simulink model "BD_INTERACTIVE_REPLAY"  (Simulink 4.00)
settings: Solver=FixedStepDiscrete  StartTime=0.0  StopTime=inf  FixedStep=1  RelTol=1e-3
undefined symbols (not defined in the file): fc_plot_axis, mc_plot_axis
libraries: lib_interactive x1
settings Model: LastModifiedBy=mokeefe  LimitDataPoints=off  ExtModeTrigMode=oneshot  ExtModeArmWhenConnect=off
settings Model: ModifiedComment=|
  | mokeefe -- Thu Apr 18 07:59:04 2002 -- Version 1.86
  | saving the model:
  | o "without the model browser open"
  | o with only top-level screen visible
  | o and with "fit to view" enabled
settings Model: ModifiedHistory=|
  | mokeefe -- Thu Apr 18 07:59:04 2002 -- Version 1.86
  | saving the model:
  | o "without the model browser open"
  | o with only top-level screen visible
  | o and with "fit to view" enabled

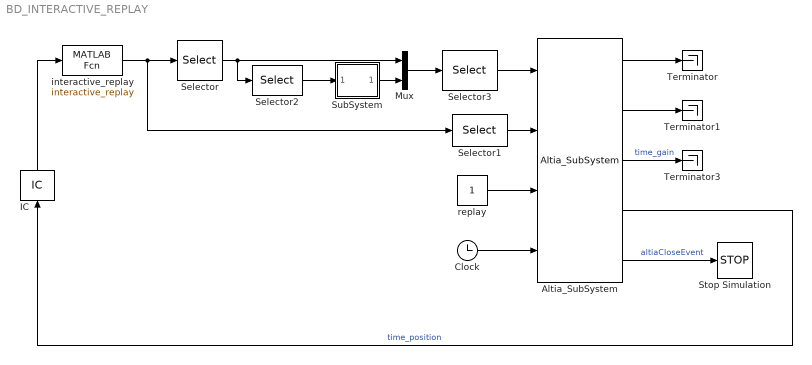
== system BD_INTERACTIVE_REPLAY ==
  Altia_SubSystem : lib_interactive/Altia_SubSystem
      settings: RTWFcnNameOpts=Auto  RTWFileNameOpts=Auto
  Clock : Clock
      settings: DisplayTime=off  Decimation=10
  IC : InitialCondition  Orientation=up  Value=1
  Mux : Mux  Inputs=2
  Selector : Selector  InputType=Vector  ElementSrc=Internal  Elements=[2:47 60 49:59]  RowSrc=Internal  Rows=1  ColumnSrc=Internal  Columns=1  InputPortWidth=60
  Selector1 : Selector  InputType=Vector  ElementSrc=Internal  Elements=[1]  RowSrc=Internal  Rows=1  ColumnSrc=Internal  Columns=1  InputPortWidth=60
  Selector2 : Selector  InputType=Vector  ElementSrc=Internal  Elements=[22 23 56 57 58]  RowSrc=Internal  Rows=1  ColumnSrc=Internal  Columns=1  InputPortWidth=58
  Selector3 : Selector  InputType=Vector  ElementSrc=Internal  Elements=[1:28 59 60 31:52 61 62 63 56:58]  RowSrc=Internal  Rows=1  ColumnSrc=Internal  Columns=1  InputPortWidth=63
  Stop Simulation : Stop
  SubSystem : Subsystem
      settings: RTWFcnNameOpts=Auto  RTWFileNameOpts=Auto
  Terminator : Terminator
  Terminator1 : Terminator
  Terminator3 : Terminator
  interactive_replay : MATLABFcn  MATLABFcn=interactive_replay  OutputDimensions=60  OutputSignalType=auto  Output1D=on
  replay : Constant  Value=1
  wires:
  interactive_replay/1 -> Selector/1, Selector1/1
  Altia_SubSystem/1 -> Terminator/1
  Altia_SubSystem/2 -> Terminator1/1
  replay/1 -> Altia_SubSystem/3
  Altia_SubSystem/3 -> Terminator3/1  "time_gain"
  Clock/1 -> Altia_SubSystem/4
  Altia_SubSystem/5 -> Stop Simulation/1  "altiaCloseEvent"
  Selector1/1 -> Altia_SubSystem/2
  Selector3/1 -> Altia_SubSystem/1
  Selector/1 -> Selector2/1, Mux/1
  Mux/1 -> Selector3/1
  Selector2/1 -> SubSystem/1(In1)
  SubSystem/1(Out1) -> Mux/2
  IC/1 -> interactive_replay/1
  Altia_SubSystem/4 -> IC/1  "time_position"

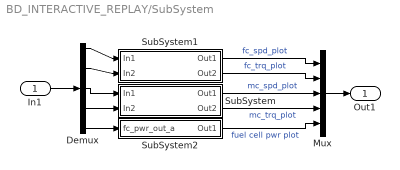
== system BD_INTERACTIVE_REPLAY/SubSystem ==
  In1 : Inport  Port=1  LatchInput=off
  Demux : Demux  Outputs=5  BusSelectionMode=off
  Mux : Mux  Inputs=5
  SubSystem : Subsystem
      settings: RTWFcnNameOpts=Auto  RTWFileNameOpts=Auto
  SubSystem1 : Subsystem
      settings: RTWFcnNameOpts=Auto  RTWFileNameOpts=Auto
  SubSystem2 : Subsystem
      settings: RTWFcnNameOpts=Auto  RTWFileNameOpts=Auto
  Out1 : Outport  Port=1
  wires:
  In1/1 -> Demux/1
  Demux/1 -> SubSystem1/1(In1)
  Demux/2 -> SubSystem1/2(In2)
  Demux/3 -> SubSystem/1(In1)
  Demux/4 -> SubSystem/2(In2)
  SubSystem/1(Out1) -> Mux/3  "mc_spd_plot"
  SubSystem/2(Out2) -> Mux/4  "mc_trq_plot"
  SubSystem1/1(Out1) -> Mux/1  "fc_spd_plot"
  SubSystem1/2(Out2) -> Mux/2  "fc_trq_plot"
  Mux/1 -> Out1/1
  SubSystem2/1(Out1) -> Mux/5  "fuel cell pwr plot"
  Demux/5 -> SubSystem2/1(fc_pwr_out_a)

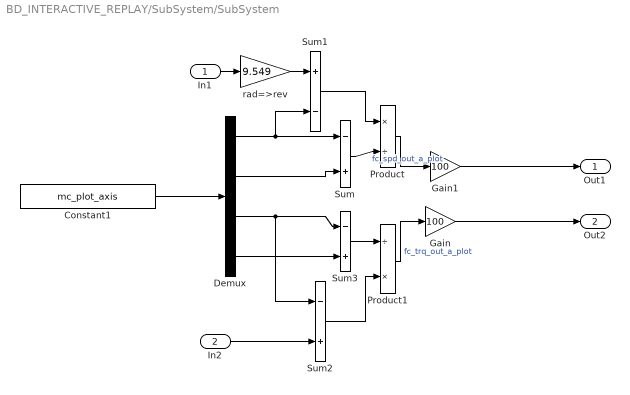
== system BD_INTERACTIVE_REPLAY/SubSystem/SubSystem ==
  In1 : Inport  Port=1  LatchInput=off
  In2 : Inport  Port=2  LatchInput=off
  Constant1 : Constant  Value=mc_plot_axis
  Demux : Demux  Outputs=4  BusSelectionMode=off
  Gain : Gain  Gain=100  Multiplication=Element-wise(K.*u)  SaturateOnIntegerOverflow=on
  Gain1 : Gain  Gain=100  Multiplication=Element-wise(K.*u)  SaturateOnIntegerOverflow=on
  Product : Product  Inputs=*/  Multiplication=Element-wise(.*)  SaturateOnIntegerOverflow=on
  Product1 : Product  Inputs=/*  Multiplication=Element-wise(.*)  SaturateOnIntegerOverflow=on
  Sum : Sum  Inputs=-+  SaturateOnIntegerOverflow=on
  Sum1 : Sum  Inputs=+-  SaturateOnIntegerOverflow=on
  Sum2 : Sum  Inputs=-+  SaturateOnIntegerOverflow=on
  Sum3 : Sum  Inputs=-+  SaturateOnIntegerOverflow=on
  rad=>rev : Gain  Gain=9.549  Multiplication=Element-wise(K.*u)  SaturateOnIntegerOverflow=on
  Out1 : Outport  Port=1
  Out2 : Outport  Port=2
  wires:
  Gain/1 -> Out2/1
  Gain1/1 -> Out1/1
  Product/1 -> Gain1/1  "fc_spd_out_a_plot"
  Product1/1 -> Gain/1  "fc_trq_out_a_plot"
  Demux/3 -> Sum2/1, Sum3/1
  Demux/4 -> Sum3/2
  Sum2/1 -> Product1/2
  Sum3/1 -> Product1/1
  Sum1/1 -> Product/1
  Demux/1 -> Sum1/2, Sum/1
  Sum/1 -> Product/2
  Demux/2 -> Sum/2
  Constant1/1 -> Demux/1
  In2/1 -> Sum2/2
  In1/1 -> rad=>rev/1
  rad=>rev/1 -> Sum1/1

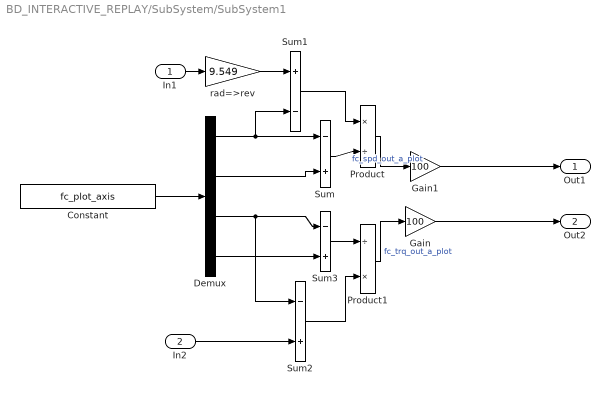
== system BD_INTERACTIVE_REPLAY/SubSystem/SubSystem1 ==
  In1 : Inport  Port=1  LatchInput=off
  In2 : Inport  Port=2  LatchInput=off
  Constant : Constant  Value=fc_plot_axis
  Demux : Demux  Outputs=4  BusSelectionMode=off
  Gain : Gain  Gain=100  Multiplication=Element-wise(K.*u)  SaturateOnIntegerOverflow=on
  Gain1 : Gain  Gain=100  Multiplication=Element-wise(K.*u)  SaturateOnIntegerOverflow=on
  Product : Product  Inputs=*/  Multiplication=Element-wise(.*)  SaturateOnIntegerOverflow=on
  Product1 : Product  Inputs=/*  Multiplication=Element-wise(.*)  SaturateOnIntegerOverflow=on
  Sum : Sum  Inputs=-+  SaturateOnIntegerOverflow=on
  Sum1 : Sum  Inputs=+-  SaturateOnIntegerOverflow=on
  Sum2 : Sum  Inputs=-+  SaturateOnIntegerOverflow=on
  Sum3 : Sum  Inputs=-+  SaturateOnIntegerOverflow=on
  rad=>rev : Gain  Gain=9.549  Multiplication=Element-wise(K.*u)  SaturateOnIntegerOverflow=on
  Out1 : Outport  Port=1
  Out2 : Outport  Port=2
  wires:
  Demux/2 -> Sum/2
  Sum/1 -> Product/2
  Demux/1 -> Sum/1, Sum1/2
  Sum1/1 -> Product/1
  In2/1 -> Sum2/2
  Sum3/1 -> Product1/1
  Sum2/1 -> Product1/2
  Demux/4 -> Sum3/2
  Demux/3 -> Sum3/1, Sum2/1
  Product1/1 -> Gain/1  "fc_trq_out_a_plot"
  Product/1 -> Gain1/1  "fc_spd_out_a_plot"
  Gain1/1 -> Out1/1
  Gain/1 -> Out2/1
  Constant/1 -> Demux/1
  In1/1 -> rad=>rev/1
  rad=>rev/1 -> Sum1/1

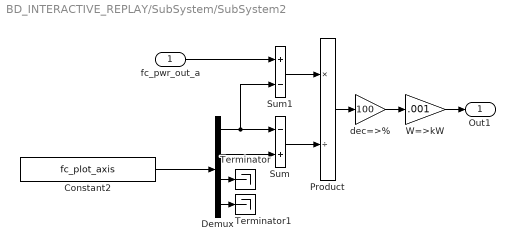
== system BD_INTERACTIVE_REPLAY/SubSystem/SubSystem2 ==
  fc_pwr_out_a : Inport  Port=1  LatchInput=off
  Constant2 : Constant  Value=fc_plot_axis
  Demux : Demux  Outputs=4  BusSelectionMode=off
  Product : Product  Inputs=*/  Multiplication=Element-wise(.*)  SaturateOnIntegerOverflow=on
  Sum : Sum  Inputs=-+  SaturateOnIntegerOverflow=on
  Sum1 : Sum  Inputs=+-  SaturateOnIntegerOverflow=on
  Terminator : Terminator
  Terminator1 : Terminator
  W=>kW : Gain  Gain=.001  Multiplication=Element-wise(K.*u)  SaturateOnIntegerOverflow=on
  dec=>% : Gain  Gain=100  Multiplication=Element-wise(K.*u)  SaturateOnIntegerOverflow=on
  Out1 : Outport  Port=1
  wires:
  Demux/3 -> Terminator/1
  Demux/4 -> Terminator1/1
  Demux/2 -> Sum/2
  Demux/1 -> Sum/1, Sum1/2
  Sum1/1 -> Product/1
  Sum/1 -> Product/2
  dec=>%/1 -> W=>kW/1
  W=>kW/1 -> Out1/1
  Product/1 -> dec=>%/1
  Constant2/1 -> Demux/1
  fc_pwr_out_a/1 -> Sum1/1
